simulink model "Three_Phase_Half_Controlled_Rectifier_RL_Load"  (R2018a)
settings: Solver=VariableStepAuto  StartTime=0.0  StopTime=0.1  RelTol=1e-3
libraries: powerlib x19, powerlib_meascontrol x5
settings Model: Creator=ozie  LastModifiedBy=ozie

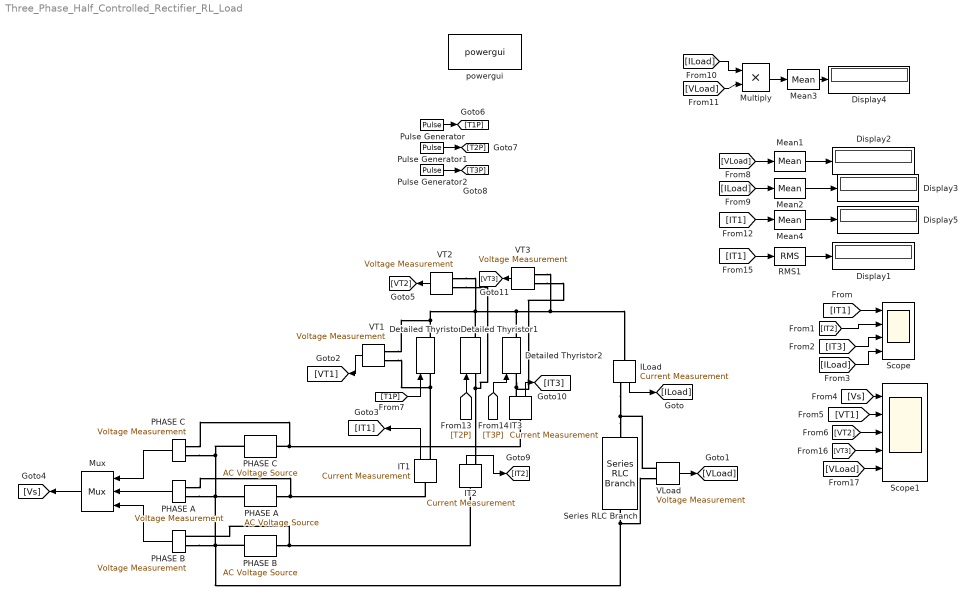
== system Three_Phase_Half_Controlled_Rectifier_RL_Load ==
  Detailed Thyristor : powerlib/Power Electronics/Detailed Thyristor  Ron=0.001  Lon=1e-3  Vf=0.8  IL=0.1  Tq=100e-6  IC=0  Rs=1e6  Cs=250e-9  Measurements=on
      settings: SourceProductName=Simscape Power Systems  SourceProductBaseCode=PS
  Detailed Thyristor1 : powerlib/Power Electronics/Detailed Thyristor  Ron=0.001  Lon=1e-3  Vf=0.8  IL=0.1  Tq=100e-6  IC=0  Rs=1e6  Cs=250e-9  Measurements=on
      settings: SourceProductName=Simscape Power Systems  SourceProductBaseCode=PS
  Detailed Thyristor2 : powerlib/Power Electronics/Detailed Thyristor  Ron=0.001  Lon=1e-3  Vf=0.8  IL=0.1  Tq=100e-6  IC=0  Rs=1e6  Cs=250e-9  Measurements=on
      settings: SourceProductName=Simscape Power Systems  SourceProductBaseCode=PS
  Display{1..5} (5 alike) : Display
      Display4 settings: Format=bank
      Display5 settings: Format=bank
  ILoad : powerlib/Measurements/Current Measurement  PhasorSimulation=off  OutputType=Complex  PSBequivalent=0
  IT1 : powerlib/Measurements/Current Measurement  PhasorSimulation=off  OutputType=Complex  PSBequivalent=0
  IT2 : powerlib/Measurements/Current Measurement  PhasorSimulation=off  OutputType=Complex  PSBequivalent=0
  IT3 : powerlib/Measurements/Current Measurement  PhasorSimulation=off  OutputType=Complex  PSBequivalent=0
  Mean{1..4} (4 alike) : powerlib_meascontrol/Measurements/Mean  Freq=50  Vinit=0  Ts=0
  Multiply : Product
  Mux : Mux  Inputs=3
      settings: DisplayOption=signals
  PHASE A : powerlib/Electrical Sources/AC Voltage Source  Amplitude=220*sqrt(2)  Phase=0  Frequency=50  SampleTime=0  Measurements=None  BusType=swing  Pref=10e3  Qref=0  Qmin=-inf  Qmax=+inf
  "PHASE A " : powerlib/Measurements/Voltage Measurement  PhasorSimulation=off  OutputType=Complex  PSBequivalent=0
  PHASE B : powerlib/Electrical Sources/AC Voltage Source  Amplitude=220*sqrt(2)  Phase=-120  Frequency=50  SampleTime=0  Measurements=None  BusType=swing  Pref=10e3  Qref=0  Qmin=-inf  Qmax=+inf
  "PHASE B " : powerlib/Measurements/Voltage Measurement  PhasorSimulation=off  OutputType=Complex  PSBequivalent=0
  PHASE C : powerlib/Measurements/Voltage Measurement  PhasorSimulation=off  OutputType=Complex  PSBequivalent=0
  "PHASE C " : powerlib/Electrical Sources/AC Voltage Source  Amplitude=220*sqrt(2)  Phase=120  Frequency=50  SampleTime=0  Measurements=None  BusType=swing  Pref=10e3  Qref=0  Qmin=-inf  Qmax=+inf
  Pulse Generator : DiscretePulseGenerator  PulseType=Time based  Period=1/50  PulseWidth=5  PhaseDelay=0.01*(120/180)
  Pulse Generator1 : DiscretePulseGenerator  PulseType=Time based  Period=1/50  PulseWidth=5  PhaseDelay=0.01*(240/180)
  Pulse Generator2 : DiscretePulseGenerator  PulseType=Time based  Period=1/50  PulseWidth=5
  RMS1 : powerlib_meascontrol/Measurements/RMS  TrueRMS=on  Freq=50  RMSInit=120  Ts=0
  Scope : Scope  NumInputPorts=4
  Scope1 : Scope  NumInputPorts=5
  Series RLC Branch : powerlib/Elements/Series RLC Branch  LConnTagsString=__new0  RConnTagsString=__new0  BranchType=RL  Resistance=100  Inductance=100e-3  SetiL0=off  InitialCurrent=0  Capacitance=1e-6  Setx0=off  InitialVoltage=0  Measurements=None
  "VLoad " : powerlib/Measurements/Voltage Measurement  PhasorSimulation=off  OutputType=Complex  PSBequivalent=0
  "VT1 " : powerlib/Measurements/Voltage Measurement  PhasorSimulation=off  OutputType=Complex  PSBequivalent=0
  VT2 : powerlib/Measurements/Voltage Measurement  PhasorSimulation=off  OutputType=Complex  PSBequivalent=0
  VT3 : powerlib/Measurements/Voltage Measurement  PhasorSimulation=off  OutputType=Complex  PSBequivalent=0
  powergui : powerlib/powergui  Priority=1  SimulationMode=Continuous  SampleTime=50e-6  frequency=60  Iterations=50  frequencyindice=50  Pbase=100e6  ErrMax=1e-4  UnitsV=kV  UnitsW=MW  buscounter=0  FunctionMessages=off  echomessages=off  EnableUseOfTLC=off  CurrentSourceSwitches=off  DisableSnubberDevices=off  DisableRonSwitches=off  DisableVfSwitches=off  DisplayEquations=off  SolverType=Tustin/Backward Euler (TBE)  Interpol=off  ExternalGateDelay=off  methode=off  Ts=100  x0status=blocks  SPID=on  SwTol=0  HookPort=off  RestoreLinks=warning  ResistiveCurrentMeasurement=off  Frange=[0:2:500]  Ylog=off  Xlog=on  ShowGrid=off  save=off  variable=ZData  structure=0  ZoomFFT=off  StartTime=0.0  cycles=1  DisplayStyle=1  fundamental=60  FreqAxis=off  MaxFrequency=1000  frequencyindicesteady=1  RmsSteady=1  display=off
  wires:
  Mux/1 -> [Vs]
  Mean2/1 -> Display3/1
  IT1/1 -> [IT1]
  Mean4/1 -> Display5/1
  "VLoad "/1 -> [VLoad]
  Multiply/1 -> Mean3/1
  ILoad/1 -> [ILoad]
  [ILoad] -> Mean2/1
  [VLoad] -> Mean1/1
  [ILoad] -> Multiply/1
  Mean3/1 -> Display4/1
  [VLoad] -> Multiply/2
  Mean1/1 -> Display2/1
  "PHASE A "/1 -> Mux/2
  "PHASE B "/1 -> Mux/3
  "VT1 "/1 -> [VT1]
  PHASE C/1 -> Mux/1
  [IT1] -> Mean4/1
  Pulse Generator/1 -> [T1P]
  Pulse Generator1/1 -> [T2P]
  Pulse Generator2/1 -> [T3P]
  [T1P] -> Detailed Thyristor/1
  [T2P] -> Detailed Thyristor1/1
  [T3P] -> Detailed Thyristor2/1
  RMS1/1 -> Display1/1
  [IT1] -> RMS1/1
  IT2/1 -> [IT2]
  IT3/1 -> [IT3]
  [IT1] -> Scope/1
  [IT2] -> Scope/2
  [IT3] -> Scope/3
  [ILoad] -> Scope/4
  VT2/1 -> [VT2]
  VT3/1 -> [VT3]
  [Vs] -> Scope1/1
  [VT1] -> Scope1/2
  [VT2] -> Scope1/3
  [VT3] -> Scope1/4
  [VLoad] -> Scope1/5
  connections:
  PHASE C/LConn2 -- "PHASE C "/LConn1 -- PHASE A/LConn1 -- "VLoad "/LConn2 -- Series RLC Branch/RConn1 -- "PHASE B "/LConn2 -- PHASE B/LConn1 -- "PHASE A "/LConn2
  Detailed Thyristor2/RConn1 -- "VT1 "/LConn2 -- Detailed Thyristor/RConn1 -- VT2/LConn2 -- Detailed Thyristor1/RConn1 -- VT3/LConn2 -- ILoad/LConn1
  Series RLC Branch/LConn1 -- ILoad/RConn1 -- "VLoad "/LConn1
  PHASE A/RConn1 -- IT1/LConn1 -- "PHASE A "/LConn1
  IT1/RConn1 -- "VT1 "/LConn1 -- Detailed Thyristor/LConn1
  IT3/RConn1 -- VT3/LConn1 -- Detailed Thyristor2/LConn1
  PHASE B/RConn1 -- IT2/LConn1 -- "PHASE B "/LConn1
  Detailed Thyristor1/LConn1 -- VT2/LConn1 -- IT2/RConn1
  PHASE C/LConn1 -- IT3/LConn1 -- "PHASE C "/RConn1
